simulink model "AI6109_MOA_AutoComp7"  (R2023b)
settings: Solver=FixedStepDiscrete  StartTime=0.0  StopTime=0.5  FixedStep=Ts  MaxStep=0.2  RelTol=1e-4  EnableMultiTasking=on
values from neighbouring files (symbols this model uses):
  f = figure('Color','w','Position',[100 100 1050 540])    [run_gating_ablation.m]    (also in run_m5_step5_robustness.m = context.dataF; run_phase2_simulink_dynamic.m = figure('Color','w','Position',[100 100 1000 520]))
undefined symbols (not defined in the file or in its folder): C0, C1, C2, C_moa, h3_ratio, phi3_deg, StopTime, Ts, Un_LL, Vneg_pu
libraries: spsSeriesRLCBranchLib x13, spsCurrentMeasurementLib x6, spsVoltageMeasurementLib x6, spsGroundLib x4, spsControlledCurrentSourceLib x3, spsThreePhaseProgrammableVoltageSourceLib x1, spspowerguiLib x1
settings Model: Creator=18423  LastModifiedBy=Administrator
settings SolverCC: AlgebraicLoopSolver=TrustRegion  MaxZcPerStep=1
settings DataIOCC: LimitDataPoints=on  MaxDataPoints=10000  ReturnWorkspaceOutputs=off
settings OptimizationCC: ReuseModelBlockBuffer=off  LifeSpan=inf
settings DebuggingCC: UnconnectedInputMsg=warning  UnconnectedOutputMsg=warning  UnconnectedLineMsg=warning  AllowSymbolicDim=off  SFUnexpectedBacktrackingDiag=warning  SFNoUnconditionalDefaultTransitionDiag=warning  SFExecutionAtInitializationDiag=none  ArithmeticOperatorsInVariantConditions=warning
settings ModelReferenceCC: EnableRefExpFcnMdlSchedulingChecks=on
settings SFSimCC: SimUseLocalCustomCode=off  CustomCodeUndefinedFunction=UseInterfaceOnly
settings RTWCC: RTWUseLocalCustomCode=off  DLArmComputeVersion=19.05
settings CodeAppCC: StateflowObjectComments=on
settings GRTTargetCC: TargetLangStandard=C89/C90 (ANSI)
settings ConfigComp: CovMetricSettings=dw  CovSaveCumulativeToWorkspaceVar=on  CovSaveSingleToWorkspaceVar=on  CovExternalEMLEnable=off  CovSFcnEnable=off
settings SimscapeCC: SimscapeLogType=all  SimscapeLogDataHistory=10000

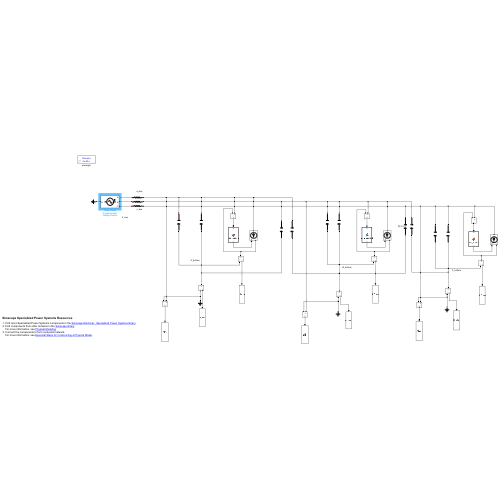
[thumbnail: Simulink's stored preview of the top-level diagram]
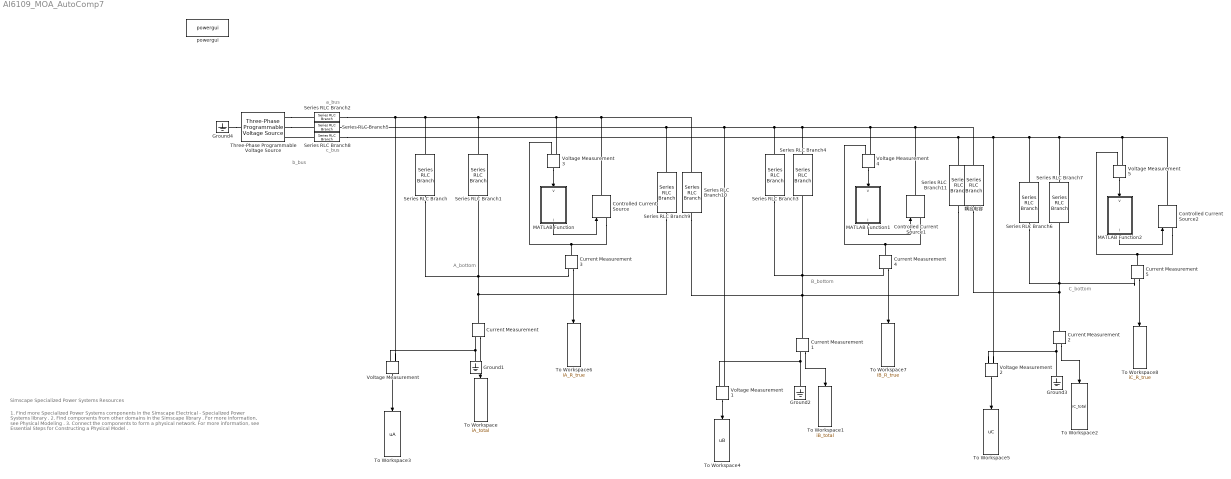
== system AI6109_MOA_AutoComp7 ==
  note: A_bottom
  note: c_bus
  note: b_bus
  note: a_bus
  note: 1. Find more Specialized Power Systems components in the Simscape Electrical - Specialized Power Systems library .
      | 2. Find components from other domains in the Simscape library .
      | For more information, see Physical Modeling .
      | 3. Connect the components to form a physical network.
      | For more information, see Essential Steps for Constructing a Physical Model .
  note: Simscape Specialized Power Systems Resources
  note: B_bottom
  note: C_bottom
  Controlled Current Source : spsControlledCurrentSourceLib/Controlled Current Source  Initialize=on  Source_Type=AC  Amplitude=0  Phase=0  Frequency=0  Measurements=None
  Controlled Current Source1 : spsControlledCurrentSourceLib/Controlled Current Source  Initialize=on  Source_Type=AC  Amplitude=0  Phase=0  Frequency=0  Measurements=None
  Controlled Current Source2 : spsControlledCurrentSourceLib/Controlled Current Source  Initialize=on  Source_Type=AC  Amplitude=0  Phase=0  Frequency=0  Measurements=None
  Current Measurement{,1..5} (6 alike) : spsCurrentMeasurementLib/Current Measurement  PhasorSimulation=off  OutputType=Complex  PSBequivalent=0
  Ground{1..4} (4 alike) : spsGroundLib/Ground  LConnTagsString=a
  MATLAB Function : MATLAB Function  TreatAsAtomicUnit=on
  MATLAB Function1 : MATLAB Function  TreatAsAtomicUnit=on
  MATLAB Function2 : MATLAB Function  TreatAsAtomicUnit=on
  Series RLC Branch : spsSeriesRLCBranchLib/Series RLC Branch  LConnTagsString=__new0  RConnTagsString=__new0  BranchType=C  Resistance=1  Inductance=1e-3  SetiL0=off  InitialCurrent=0  Capacitance=C0  Setx0=off  InitialVoltage=0  Measurements=None
  Series RLC Branch1 : spsSeriesRLCBranchLib/Series RLC Branch  LConnTagsString=__new0  RConnTagsString=__new0  BranchType=C  Resistance=1  Inductance=1e-3  SetiL0=off  InitialCurrent=0  Capacitance=C_moa  Setx0=off  InitialVoltage=0  Measurements=None
  Series RLC Branch10 : spsSeriesRLCBranchLib/Series RLC Branch  LConnTagsString=__new0  RConnTagsString=__new0  BranchType=C  Resistance=1  Inductance=1e-3  SetiL0=off  InitialCurrent=0  Capacitance=C1  Setx0=off  InitialVoltage=0  Measurements=None
  Series RLC Branch11 : spsSeriesRLCBranchLib/Series RLC Branch  LConnTagsString=__new0  RConnTagsString=__new0  BranchType=C  Resistance=1  Inductance=1e-3  SetiL0=off  InitialCurrent=0  Capacitance=C2  Setx0=off  InitialVoltage=0  Measurements=None
  Series RLC Branch2 : spsSeriesRLCBranchLib/Series RLC Branch  LConnTagsString=__new0  RConnTagsString=__new0  BranchType=R  Resistance=0.1  Inductance=1e-3  SetiL0=off  InitialCurrent=0  Capacitance=C_moa  Setx0=off  InitialVoltage=0  Measurements=None
  Series RLC Branch3 : spsSeriesRLCBranchLib/Series RLC Branch  LConnTagsString=__new0  RConnTagsString=__new0  BranchType=C  Resistance=1  Inductance=1e-3  SetiL0=off  InitialCurrent=0  Capacitance=C0  Setx0=off  InitialVoltage=0  Measurements=None
  Series RLC Branch4 : spsSeriesRLCBranchLib/Series RLC Branch  LConnTagsString=__new0  RConnTagsString=__new0  BranchType=C  Resistance=1  Inductance=1e-3  SetiL0=off  InitialCurrent=0  Capacitance=C_moa  Setx0=off  InitialVoltage=0  Measurements=None
  Series RLC Branch5 : spsSeriesRLCBranchLib/Series RLC Branch  LConnTagsString=__new0  RConnTagsString=__new0  BranchType=R  Resistance=0.1  Inductance=1e-3  SetiL0=off  InitialCurrent=0  Capacitance=C_moa  Setx0=off  InitialVoltage=0  Measurements=None
  Series RLC Branch6 : spsSeriesRLCBranchLib/Series RLC Branch  LConnTagsString=__new0  RConnTagsString=__new0  BranchType=C  Resistance=1  Inductance=1e-3  SetiL0=off  InitialCurrent=0  Capacitance=C0  Setx0=off  InitialVoltage=0  Measurements=None
  Series RLC Branch7 : spsSeriesRLCBranchLib/Series RLC Branch  LConnTagsString=__new0  RConnTagsString=__new0  BranchType=C  Resistance=1  Inductance=1e-3  SetiL0=off  InitialCurrent=0  Capacitance=C_moa  Setx0=off  InitialVoltage=0  Measurements=None
  Series RLC Branch8 : spsSeriesRLCBranchLib/Series RLC Branch  LConnTagsString=__new0  RConnTagsString=__new0  BranchType=R  Resistance=0.1  Inductance=1e-3  SetiL0=off  InitialCurrent=0  Capacitance=C_moa  Setx0=off  InitialVoltage=0  Measurements=None
  Series RLC Branch9 : spsSeriesRLCBranchLib/Series RLC Branch  LConnTagsString=__new0  RConnTagsString=__new0  BranchType=C  Resistance=1  Inductance=1e-3  SetiL0=off  InitialCurrent=0  Capacitance=C1  Setx0=off  InitialVoltage=0  Measurements=None
  Three-Phase Programmable Voltage Source : spsThreePhaseProgrammableVoltageSourceLib/Three-Phase Programmable Voltage Source  PositiveSequence="[Un_LL  120 f]"  VariationEntity=None  VariationType=Table of time-amplitude pairs  VariationTypeAlt=Step  VariationStep=0.5  VariationRate=10  VariationMagnitude=0.3  VariationFrequency=2  VariationTiming=[1 2]  VariationPhaseA=off  Amplitudes=[1 0.8 1.2 1.0]  TimeValues=[0 0.1 0.15 0.2]  HarmonicGeneration=on  HarmonicA=[3 h3_ratio phi3_deg 0]  HarmonicB=[1 Vneg_pu 0 2]  Timing="[0  StopTime]"  BusType=swing  Pref=0  Qref=0  Qmin=-inf  Qmax=inf
  To Workspace : ToWorkspace  VariableName=iA_total  SaveFormat=Structure With Time  SampleTime=-1
  To Workspace1 : ToWorkspace  VariableName=iB_total  SaveFormat=Structure With Time  SampleTime=-1
  To Workspace2 : ToWorkspace  VariableName=iC_total  SaveFormat=Structure With Time  SampleTime=-1
  To Workspace3 : ToWorkspace  VariableName=uA  SaveFormat=Structure With Time  SampleTime=-1
  To Workspace4 : ToWorkspace  VariableName=uB  SaveFormat=Structure With Time  SampleTime=-1
  To Workspace5 : ToWorkspace  VariableName=uC  SaveFormat=Structure With Time  SampleTime=-1
  To Workspace6 : ToWorkspace  VariableName=iA_R_true  SaveFormat=Structure With Time  SampleTime=-1
  To Workspace7 : ToWorkspace  VariableName=iB_R_true  SaveFormat=Structure With Time  SampleTime=-1
  To Workspace8 : ToWorkspace  VariableName=iC_R_true  SaveFormat=Structure With Time  SampleTime=-1
  Voltage Measurement{,1..5} (6 alike) : spsVoltageMeasurementLib/Voltage Measurement  PhasorSimulation=off  OutputType=Complex  PSBequivalent=0
  powergui : spspowerguiLib/powergui  Priority=1  SimulationMode=Discrete  SampleTime=Ts  frequency=60  Iterations=50  frequencyindice=50  Pbase=100e6  ErrMax=1e-4  UnitsV=kV  UnitsW=MW  buscounter=0  FunctionMessages=off  echomessages=off  EnableUseOfTLC=off  CurrentSourceSwitches=off  DisableSnubberDevices=off  DisableRonSwitches=off  DisableVfSwitches=off  DisplayEquations=off  AutomaticDiscreteSolvers=off  SolverType=Tustin/Backward Euler (TBE)  Interpol=off  ExternalGateDelay=off  methode=off  Ts=100  x0status=blocks  SPID=on  SwTol=0  HookPort=off  NonlinearTolerance=0  nMaxIteration=15  ContinueOnMaxIteration=off  RestoreLinks=warning  ResistiveCurrentMeasurement=off  Frange=[0:2:500]  Ylog=off  Xlog=on  ShowGrid=off  save=off  variable=ZData  structure=0  ZoomFFT=off  StartTime=0.0  cycles=1  DisplayStyle=1  fundamental=60  FreqAxis=off  MaxFrequency=1000  frequencyindicesteady=1  RmsSteady=1  display=off
  耦合电容 : spsSeriesRLCBranchLib/Series RLC Branch  LConnTagsString=__new0  RConnTagsString=__new0  BranchType=C  Resistance=1  Inductance=1e-3  SetiL0=off  InitialCurrent=0  Capacitance=C2  Setx0=off  InitialVoltage=0  Measurements=None
  wires:
  Current Measurement/1 -> To Workspace/1
  Current Measurement1/1 -> To Workspace1/1
  Current Measurement2/1 -> To Workspace2/1
  Voltage Measurement/1 -> To Workspace3/1
  Voltage Measurement1/1 -> To Workspace4/1
  Voltage Measurement2/1 -> To Workspace5/1
  Current Measurement3/1 -> To Workspace6/1
  Current Measurement4/1 -> To Workspace7/1
  Current Measurement5/1 -> To Workspace8/1
  Voltage Measurement3/1 -> MATLAB Function/1(v)
  MATLAB Function/1(i) -> Controlled Current Source/1
  MATLAB Function1/1(i) -> Controlled Current Source1/1
  Voltage Measurement4/1 -> MATLAB Function1/1(v)
  MATLAB Function2/1(i) -> Controlled Current Source2/1
  Voltage Measurement5/1 -> MATLAB Function2/1(v)
  connections:
  Controlled Current Source/RConn1 -- Series RLC Branch10/LConn1 -- Voltage Measurement3/LConn1 -- Series RLC Branch1/LConn1 -- Series RLC Branch2/RConn1 -- Voltage Measurement/LConn1 -- Series RLC Branch/LConn1
  Series RLC Branch/RConn1 -- Current Measurement3/RConn1 -- Series RLC Branch9/RConn1 -- Current Measurement/LConn1 -- Series RLC Branch1/RConn1
  Ground1/LConn1 -- Current Measurement/RConn1 -- Voltage Measurement/LConn2
  Series RLC Branch3/RConn1 -- Series RLC Branch10/RConn1 -- Series RLC Branch11/RConn1 -- Current Measurement1/LConn1 -- Current Measurement4/RConn1 -- Series RLC Branch4/RConn1
  Series RLC Branch9/LConn1 -- Controlled Current Source1/RConn1 -- 耦合电容/LConn1 -- Voltage Measurement4/LConn1 -- Series RLC Branch4/LConn1 -- Series RLC Branch3/LConn1 -- Voltage Measurement1/LConn1 -- Series RLC Branch5/RConn1
  Ground2/LConn1 -- Voltage Measurement1/LConn2 -- Current Measurement1/RConn1
  Series RLC Branch6/RConn1 -- Series RLC Branch7/RConn1 -- Current Measurement5/RConn1 -- Current Measurement2/LConn1 -- 耦合电容/RConn1
  Series RLC Branch11/LConn1 -- Series RLC Branch8/RConn1 -- Voltage Measurement2/LConn1 -- Voltage Measurement5/LConn1 -- Controlled Current Source2/RConn1 -- Series RLC Branch7/LConn1 -- Series RLC Branch6/LConn1
  Ground3/LConn1 -- Voltage Measurement2/LConn2 -- Current Measurement2/RConn1
  Controlled Current Source/LConn1 -- Current Measurement3/LConn1 -- Voltage Measurement3/LConn2
  Controlled Current Source1/LConn1 -- Current Measurement4/LConn1 -- Voltage Measurement4/LConn2
  Controlled Current Source2/LConn1 -- Current Measurement5/LConn1 -- Voltage Measurement5/LConn2
  Ground4/LConn1 -- Three-Phase Programmable Voltage Source/LConn1
  Three-Phase Programmable Voltage Source/RConn1 -- Series RLC Branch2/LConn1
  Three-Phase Programmable Voltage Source/RConn2 -- Series RLC Branch5/LConn1
  Series RLC Branch8/LConn1 -- Three-Phase Programmable Voltage Source/RConn3

== matlab function AI6109_MOA_AutoComp7/MATLAB Function ==
  data: v input; i output
function i = moa_current(v)
% 氧化锌避雷器非线性阻性电流模型
% v: 避雷器两端瞬时电压
% i: 阻性泄漏电流

Vref = 110e3/sqrt(3);   % 按实际系统相电压改
Iref = 0.3e-3;          % 额定运行电压下阻性电流，来自厂家或试验数据
alpha = 6;              % 非线性指数，来自V-I曲线，不要为拟合现场数据乱调

i = Iref * sign(v) * (abs(v)/Vref)^alpha;
end

== matlab function AI6109_MOA_AutoComp7/MATLAB Function2 ==
  data: v input; i output
function i = moa_current(v)
% 氧化锌避雷器非线性阻性电流模型
% v: 避雷器两端瞬时电压
% i: 阻性泄漏电流

Vref = 110e3/sqrt(3);   % 按实际系统相电压改
Iref = 0.3e-3;          % 额定运行电压下阻性电流，来自厂家或试验数据
alpha = 6;              % 非线性指数，来自V-I曲线，不要为拟合现场数据乱调

i = Iref * sign(v) * (abs(v)/Vref)^alpha;
end

== matlab function AI6109_MOA_AutoComp7/MATLAB Function1 ==
  data: v input; i output
function i = moa_current(v)
% 氧化锌避雷器非线性阻性电流模型
% v: 避雷器两端瞬时电压
% i: 阻性泄漏电流

Vref = 110e3/sqrt(3);   % 按实际系统相电压改
Iref = 0.3e-3;          % 额定运行电压下阻性电流，来自厂家或试验数据
alpha = 6;              % 非线性指数，来自V-I曲线，不要为拟合现场数据乱调

i = Iref * sign(v) * (abs(v)/Vref)^alpha;
end
